simulink model "fourbitserialadder"  (R2023a)
settings: Solver=VariableStepAuto  StartTime=0.0  StopTime=10  RelTol=1e-3
libraries: simulink_extras x12
settings Model: Creator=prath  LastModifiedBy=prath

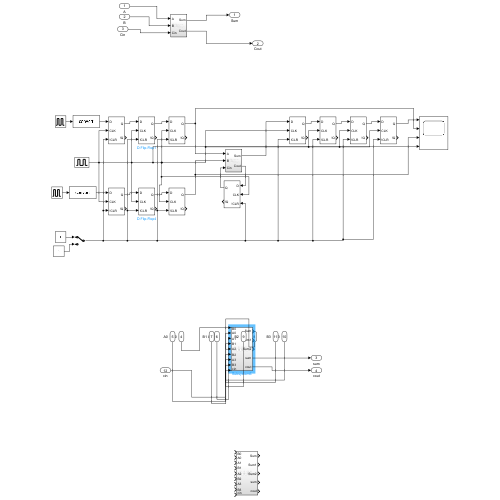
[thumbnail: Simulink's stored preview of the top-level diagram]
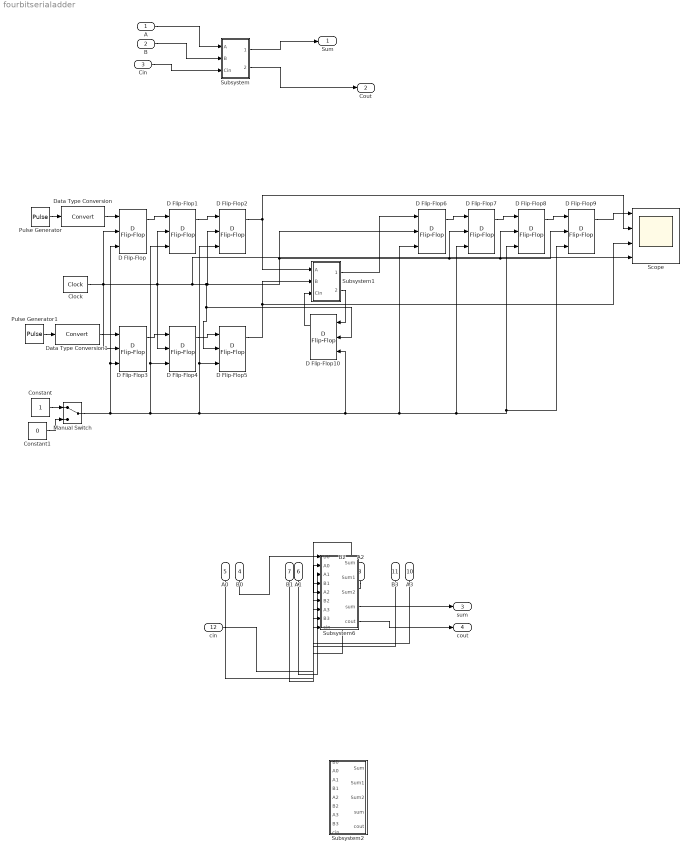
== system fourbitserialadder ==
  A : Inport
  B : Inport  Port=2
  Cin : Inport  Port=3
  B0 : Inport  Port=4
  A0 : Inport  Port=5
  A1 : Inport  Port=6
  B1 : Inport  Port=7
  A2 : Inport  Port=8
  B2 : Inport  Port=9
  A3 : Inport  Port=10
  B3 : Inport  Port=11
  cin : Inport  Port=12
  Clock : simulink_extras/Flip Flops/Clock  period=0.5
  Constant : Constant
  Constant1 : Constant  Value=0
  D Flip-Flop{,1..10} (11 alike) : simulink_extras/Flip Flops/D Flip-Flop
  Data Type Conversion : DataTypeConversion  SaturateOnIntegerOverflow=off  RndMeth=Floor
  Data Type Conversion1 : DataTypeConversion  SaturateOnIntegerOverflow=off  RndMeth=Floor
  Manual Switch : ManualSwitch
  Pulse Generator : DiscretePulseGenerator  PulseType=Time based  PulseWidth=50
  Pulse Generator1 : DiscretePulseGenerator  PulseType=Time based  Period=1  PulseWidth=50
  Scope : Scope  NumInputPorts=4
  Subsystem : Subsystem
  Subsystem1 : Subsystem
  Subsystem2 : Subsystem
  Subsystem6 : Subsystem
  Sum : Outport
  Cout : Outport  Port=2
  sum : Outport  Port=3
  cout : Outport  Port=4
  wires:
  A/1 -> Subsystem/1(A)
  B/1 -> Subsystem/2(B)
  Cin/1 -> Subsystem/3(Cin)
  Subsystem/1(Sum) -> Sum/1
  Subsystem/2(Cout) -> Cout/1
  D Flip-Flop/1 -> D Flip-Flop1/1
  D Flip-Flop1/1 -> D Flip-Flop2/1
  D Flip-Flop3/1 -> D Flip-Flop4/1
  D Flip-Flop4/1 -> D Flip-Flop5/1
  Subsystem1/2(Cout) -> D Flip-Flop10/1
  D Flip-Flop10/1 -> Subsystem1/3(Cin)
  Subsystem1/1(Sum) -> D Flip-Flop6/1
  D Flip-Flop6/1 -> D Flip-Flop7/1
  D Flip-Flop7/1 -> D Flip-Flop8/1
  D Flip-Flop8/1 -> D Flip-Flop9/1
  Clock/1 -> D Flip-Flop3/2, D Flip-Flop4/2, Scope/4, D Flip-Flop9/2, D Flip-Flop8/2, D Flip-Flop7/2, D Flip-Flop6/2, D Flip-Flop2/2, D Flip-Flop10/2, D Flip-Flop5/2, D Flip-Flop1/2, D Flip-Flop/2
  Pulse Generator/1 -> Data Type Conversion/1
  Data Type Conversion/1 -> D Flip-Flop/1
  Pulse Generator1/1 -> Data Type Conversion1/1
  Data Type Conversion1/1 -> D Flip-Flop3/1
  Constant/1 -> Manual Switch/1
  Constant1/1 -> Manual Switch/2
  Manual Switch/1 -> D Flip-Flop3/3, D Flip-Flop/3, D Flip-Flop4/3, D Flip-Flop1/3, D Flip-Flop10/3, D Flip-Flop9/3, D Flip-Flop8/3, D Flip-Flop7/3, D Flip-Flop6/3, D Flip-Flop5/3, D Flip-Flop2/3
  D Flip-Flop2/1 -> Subsystem1/1(A), Scope/2
  D Flip-Flop5/1 -> Scope/3, Subsystem1/2(B)
  D Flip-Flop9/1 -> Scope/1
  B0/1 -> Subsystem6/1(B0)
  A0/1 -> Subsystem6/2(A0)
  A1/1 -> Subsystem6/3(A1)
  B1/1 -> Subsystem6/4(B1)
  A2/1 -> Subsystem6/5(A2)
  B2/1 -> Subsystem6/6(B2)
  A3/1 -> Subsystem6/7(A3)
  B3/1 -> Subsystem6/8(B3)
  cin/1 -> Subsystem6/9(cin)
  Subsystem6/4(sum) -> sum/1
  Subsystem6/5(cout) -> cout/1

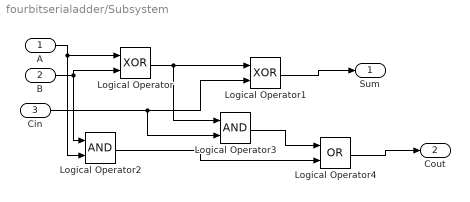
== system fourbitserialadder/Subsystem ==
  A : Inport
  B : Inport  Port=2
  Cin : Inport  Port=3
  Logical Operator : Logic  Operator=XOR  AllPortsSameDT=off  OutDataTypeStr=boolean
  Logical Operator1 : Logic  Operator=XOR  AllPortsSameDT=off  OutDataTypeStr=boolean
  Logical Operator2 : Logic  AllPortsSameDT=off  OutDataTypeStr=boolean
  Logical Operator3 : Logic  AllPortsSameDT=off  OutDataTypeStr=boolean
  Logical Operator4 : Logic  Operator=OR  AllPortsSameDT=off  OutDataTypeStr=boolean
  Sum : Outport
  Cout : Outport  Port=2
  wires:
  B/1 -> Logical Operator/2, Logical Operator2/1
  Cin/1 -> Logical Operator3/2, Logical Operator1/2
  Logical Operator3/1 -> Logical Operator4/1
  Logical Operator2/1 -> Logical Operator4/2
  A/1 -> Logical Operator/1, Logical Operator2/2
  Logical Operator/1 -> Logical Operator3/1, Logical Operator1/1
  Logical Operator1/1 -> Sum/1
  Logical Operator4/1 -> Cout/1

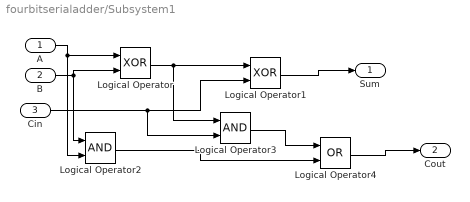
== system fourbitserialadder/Subsystem1 ==
  A : Inport
  B : Inport  Port=2
  Cin : Inport  Port=3
  Logical Operator : Logic  Operator=XOR  AllPortsSameDT=off  OutDataTypeStr=boolean
  Logical Operator1 : Logic  Operator=XOR  AllPortsSameDT=off  OutDataTypeStr=boolean
  Logical Operator2 : Logic  AllPortsSameDT=off  OutDataTypeStr=boolean
  Logical Operator3 : Logic  AllPortsSameDT=off  OutDataTypeStr=boolean
  Logical Operator4 : Logic  Operator=OR  AllPortsSameDT=off  OutDataTypeStr=boolean
  Sum : Outport
  Cout : Outport  Port=2
  wires:
  B/1 -> Logical Operator/2, Logical Operator2/1
  Cin/1 -> Logical Operator3/2, Logical Operator1/2
  Logical Operator3/1 -> Logical Operator4/1
  Logical Operator2/1 -> Logical Operator4/2
  A/1 -> Logical Operator/1, Logical Operator2/2
  Logical Operator/1 -> Logical Operator3/1, Logical Operator1/1
  Logical Operator1/1 -> Sum/1
  Logical Operator4/1 -> Cout/1

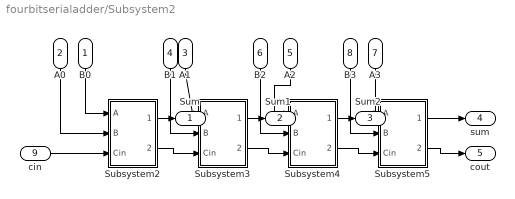
== system fourbitserialadder/Subsystem2 ==
  B0 : Inport
  A0 : Inport  Port=2
  A1 : Inport  Port=3
  B1 : Inport  Port=4
  A2 : Inport  Port=5
  B2 : Inport  Port=6
  A3 : Inport  Port=7
  B3 : Inport  Port=8
  cin : Inport  Port=9
  Subsystem2 : Subsystem
  Subsystem3 : Subsystem
  Subsystem4 : Subsystem
  Subsystem5 : Subsystem
  Sum : Outport
  Sum1 : Outport  Port=2
  Sum2 : Outport  Port=3
  sum : Outport  Port=4
  cout : Outport  Port=5
  wires:
  B0/1 -> Subsystem2/1(A)
  A2/1 -> Subsystem4/1(A)
  Subsystem2/1(Sum) -> Sum/1
  A3/1 -> Subsystem5/1(A)
  Subsystem4/1(Sum) -> Sum2/1
  cin/1 -> Subsystem2/3(Cin)
  B1/1 -> Subsystem3/2(B)
  Subsystem5/1(Sum) -> sum/1
  B2/1 -> Subsystem4/2(B)
  Subsystem5/2(Cout) -> cout/1
  B3/1 -> Subsystem5/2(B)
  Subsystem2/2(Cout) -> Subsystem3/3(Cin)
  Subsystem3/2(Cout) -> Subsystem4/3(Cin)
  Subsystem4/2(Cout) -> Subsystem5/3(Cin)
  A1/1 -> Subsystem3/1(A)
  A0/1 -> Subsystem2/2(B)
  Subsystem3/1(Sum) -> Sum1/1

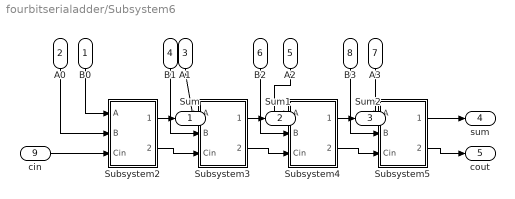
== system fourbitserialadder/Subsystem6 ==
  B0 : Inport
  A0 : Inport  Port=2
  A1 : Inport  Port=3
  B1 : Inport  Port=4
  A2 : Inport  Port=5
  B2 : Inport  Port=6
  A3 : Inport  Port=7
  B3 : Inport  Port=8
  cin : Inport  Port=9
  Subsystem2 : Subsystem
  Subsystem3 : Subsystem
  Subsystem4 : Subsystem
  Subsystem5 : Subsystem
  Sum : Outport
  Sum1 : Outport  Port=2
  Sum2 : Outport  Port=3
  sum : Outport  Port=4
  cout : Outport  Port=5
  wires:
  B0/1 -> Subsystem2/1(A)
  A2/1 -> Subsystem4/1(A)
  Subsystem2/1(Sum) -> Sum/1
  A3/1 -> Subsystem5/1(A)
  Subsystem4/1(Sum) -> Sum2/1
  cin/1 -> Subsystem2/3(Cin)
  B1/1 -> Subsystem3/2(B)
  Subsystem5/1(Sum) -> sum/1
  B2/1 -> Subsystem4/2(B)
  Subsystem5/2(Cout) -> cout/1
  B3/1 -> Subsystem5/2(B)
  Subsystem2/2(Cout) -> Subsystem3/3(Cin)
  Subsystem3/2(Cout) -> Subsystem4/3(Cin)
  Subsystem4/2(Cout) -> Subsystem5/3(Cin)
  A1/1 -> Subsystem3/1(A)
  A0/1 -> Subsystem2/2(B)
  Subsystem3/1(Sum) -> Sum1/1

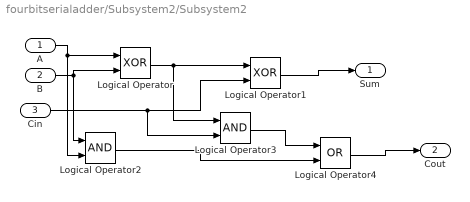
== system fourbitserialadder/Subsystem2/Subsystem2 ==
  A : Inport
  B : Inport  Port=2
  Cin : Inport  Port=3
  Logical Operator : Logic  Operator=XOR  AllPortsSameDT=off  OutDataTypeStr=boolean
  Logical Operator1 : Logic  Operator=XOR  AllPortsSameDT=off  OutDataTypeStr=boolean
  Logical Operator2 : Logic  AllPortsSameDT=off  OutDataTypeStr=boolean
  Logical Operator3 : Logic  AllPortsSameDT=off  OutDataTypeStr=boolean
  Logical Operator4 : Logic  Operator=OR  AllPortsSameDT=off  OutDataTypeStr=boolean
  Sum : Outport
  Cout : Outport  Port=2
  wires:
  B/1 -> Logical Operator/2, Logical Operator2/1
  Cin/1 -> Logical Operator3/2, Logical Operator1/2
  Logical Operator3/1 -> Logical Operator4/1
  Logical Operator2/1 -> Logical Operator4/2
  A/1 -> Logical Operator/1, Logical Operator2/2
  Logical Operator/1 -> Logical Operator3/1, Logical Operator1/1
  Logical Operator1/1 -> Sum/1
  Logical Operator4/1 -> Cout/1

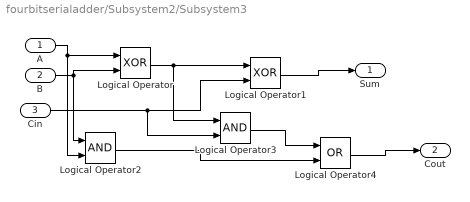
== system fourbitserialadder/Subsystem2/Subsystem3 ==
  A : Inport
  B : Inport  Port=2
  Cin : Inport  Port=3
  Logical Operator : Logic  Operator=XOR  AllPortsSameDT=off  OutDataTypeStr=boolean
  Logical Operator1 : Logic  Operator=XOR  AllPortsSameDT=off  OutDataTypeStr=boolean
  Logical Operator2 : Logic  AllPortsSameDT=off  OutDataTypeStr=boolean
  Logical Operator3 : Logic  AllPortsSameDT=off  OutDataTypeStr=boolean
  Logical Operator4 : Logic  Operator=OR  AllPortsSameDT=off  OutDataTypeStr=boolean
  Sum : Outport
  Cout : Outport  Port=2
  wires:
  B/1 -> Logical Operator/2, Logical Operator2/1
  Cin/1 -> Logical Operator3/2, Logical Operator1/2
  Logical Operator3/1 -> Logical Operator4/1
  Logical Operator2/1 -> Logical Operator4/2
  A/1 -> Logical Operator/1, Logical Operator2/2
  Logical Operator/1 -> Logical Operator3/1, Logical Operator1/1
  Logical Operator1/1 -> Sum/1
  Logical Operator4/1 -> Cout/1

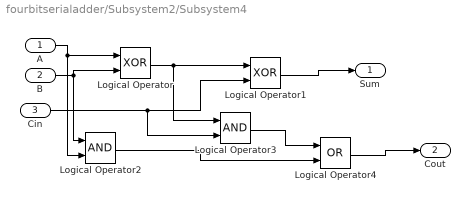
== system fourbitserialadder/Subsystem2/Subsystem4 ==
  A : Inport
  B : Inport  Port=2
  Cin : Inport  Port=3
  Logical Operator : Logic  Operator=XOR  AllPortsSameDT=off  OutDataTypeStr=boolean
  Logical Operator1 : Logic  Operator=XOR  AllPortsSameDT=off  OutDataTypeStr=boolean
  Logical Operator2 : Logic  AllPortsSameDT=off  OutDataTypeStr=boolean
  Logical Operator3 : Logic  AllPortsSameDT=off  OutDataTypeStr=boolean
  Logical Operator4 : Logic  Operator=OR  AllPortsSameDT=off  OutDataTypeStr=boolean
  Sum : Outport
  Cout : Outport  Port=2
  wires:
  B/1 -> Logical Operator/2, Logical Operator2/1
  Cin/1 -> Logical Operator3/2, Logical Operator1/2
  Logical Operator3/1 -> Logical Operator4/1
  Logical Operator2/1 -> Logical Operator4/2
  A/1 -> Logical Operator/1, Logical Operator2/2
  Logical Operator/1 -> Logical Operator3/1, Logical Operator1/1
  Logical Operator1/1 -> Sum/1
  Logical Operator4/1 -> Cout/1

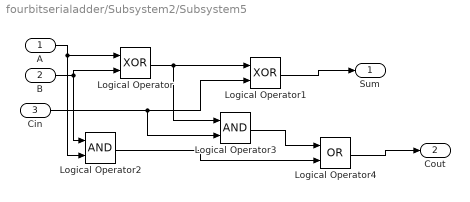
== system fourbitserialadder/Subsystem2/Subsystem5 ==
  A : Inport
  B : Inport  Port=2
  Cin : Inport  Port=3
  Logical Operator : Logic  Operator=XOR  AllPortsSameDT=off  OutDataTypeStr=boolean
  Logical Operator1 : Logic  Operator=XOR  AllPortsSameDT=off  OutDataTypeStr=boolean
  Logical Operator2 : Logic  AllPortsSameDT=off  OutDataTypeStr=boolean
  Logical Operator3 : Logic  AllPortsSameDT=off  OutDataTypeStr=boolean
  Logical Operator4 : Logic  Operator=OR  AllPortsSameDT=off  OutDataTypeStr=boolean
  Sum : Outport
  Cout : Outport  Port=2
  wires:
  B/1 -> Logical Operator/2, Logical Operator2/1
  Cin/1 -> Logical Operator3/2, Logical Operator1/2
  Logical Operator3/1 -> Logical Operator4/1
  Logical Operator2/1 -> Logical Operator4/2
  A/1 -> Logical Operator/1, Logical Operator2/2
  Logical Operator/1 -> Logical Operator3/1, Logical Operator1/1
  Logical Operator1/1 -> Sum/1
  Logical Operator4/1 -> Cout/1

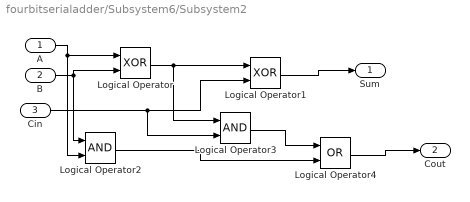
== system fourbitserialadder/Subsystem6/Subsystem2 ==
  A : Inport
  B : Inport  Port=2
  Cin : Inport  Port=3
  Logical Operator : Logic  Operator=XOR  AllPortsSameDT=off  OutDataTypeStr=boolean
  Logical Operator1 : Logic  Operator=XOR  AllPortsSameDT=off  OutDataTypeStr=boolean
  Logical Operator2 : Logic  AllPortsSameDT=off  OutDataTypeStr=boolean
  Logical Operator3 : Logic  AllPortsSameDT=off  OutDataTypeStr=boolean
  Logical Operator4 : Logic  Operator=OR  AllPortsSameDT=off  OutDataTypeStr=boolean
  Sum : Outport
  Cout : Outport  Port=2
  wires:
  B/1 -> Logical Operator/2, Logical Operator2/1
  Cin/1 -> Logical Operator3/2, Logical Operator1/2
  Logical Operator3/1 -> Logical Operator4/1
  Logical Operator2/1 -> Logical Operator4/2
  A/1 -> Logical Operator/1, Logical Operator2/2
  Logical Operator/1 -> Logical Operator3/1, Logical Operator1/1
  Logical Operator1/1 -> Sum/1
  Logical Operator4/1 -> Cout/1

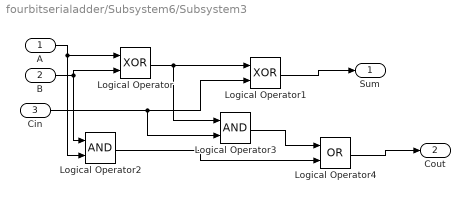
== system fourbitserialadder/Subsystem6/Subsystem3 ==
  A : Inport
  B : Inport  Port=2
  Cin : Inport  Port=3
  Logical Operator : Logic  Operator=XOR  AllPortsSameDT=off  OutDataTypeStr=boolean
  Logical Operator1 : Logic  Operator=XOR  AllPortsSameDT=off  OutDataTypeStr=boolean
  Logical Operator2 : Logic  AllPortsSameDT=off  OutDataTypeStr=boolean
  Logical Operator3 : Logic  AllPortsSameDT=off  OutDataTypeStr=boolean
  Logical Operator4 : Logic  Operator=OR  AllPortsSameDT=off  OutDataTypeStr=boolean
  Sum : Outport
  Cout : Outport  Port=2
  wires:
  B/1 -> Logical Operator/2, Logical Operator2/1
  Cin/1 -> Logical Operator3/2, Logical Operator1/2
  Logical Operator3/1 -> Logical Operator4/1
  Logical Operator2/1 -> Logical Operator4/2
  A/1 -> Logical Operator/1, Logical Operator2/2
  Logical Operator/1 -> Logical Operator3/1, Logical Operator1/1
  Logical Operator1/1 -> Sum/1
  Logical Operator4/1 -> Cout/1

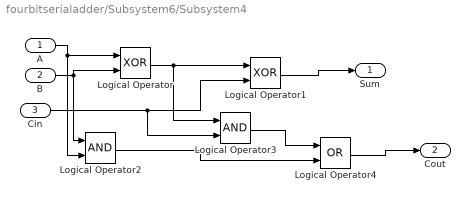
== system fourbitserialadder/Subsystem6/Subsystem4 ==
  A : Inport
  B : Inport  Port=2
  Cin : Inport  Port=3
  Logical Operator : Logic  Operator=XOR  AllPortsSameDT=off  OutDataTypeStr=boolean
  Logical Operator1 : Logic  Operator=XOR  AllPortsSameDT=off  OutDataTypeStr=boolean
  Logical Operator2 : Logic  AllPortsSameDT=off  OutDataTypeStr=boolean
  Logical Operator3 : Logic  AllPortsSameDT=off  OutDataTypeStr=boolean
  Logical Operator4 : Logic  Operator=OR  AllPortsSameDT=off  OutDataTypeStr=boolean
  Sum : Outport
  Cout : Outport  Port=2
  wires:
  B/1 -> Logical Operator/2, Logical Operator2/1
  Cin/1 -> Logical Operator3/2, Logical Operator1/2
  Logical Operator3/1 -> Logical Operator4/1
  Logical Operator2/1 -> Logical Operator4/2
  A/1 -> Logical Operator/1, Logical Operator2/2
  Logical Operator/1 -> Logical Operator3/1, Logical Operator1/1
  Logical Operator1/1 -> Sum/1
  Logical Operator4/1 -> Cout/1

== system fourbitserialadder/Subsystem6/Subsystem5 ==
  A : Inport
  B : Inport  Port=2
  Cin : Inport  Port=3
  Logical Operator : Logic  Operator=XOR  AllPortsSameDT=off  OutDataTypeStr=boolean
  Logical Operator1 : Logic  Operator=XOR  AllPortsSameDT=off  OutDataTypeStr=boolean
  Logical Operator2 : Logic  AllPortsSameDT=off  OutDataTypeStr=boolean
  Logical Operator3 : Logic  AllPortsSameDT=off  OutDataTypeStr=boolean
  Logical Operator4 : Logic  Operator=OR  AllPortsSameDT=off  OutDataTypeStr=boolean
  Sum : Outport
  Cout : Outport  Port=2
  wires:
  B/1 -> Logical Operator/2, Logical Operator2/1
  Cin/1 -> Logical Operator3/2, Logical Operator1/2
  Logical Operator3/1 -> Logical Operator4/1
  Logical Operator2/1 -> Logical Operator4/2
  A/1 -> Logical Operator/1, Logical Operator2/2
  Logical Operator/1 -> Logical Operator3/1, Logical Operator1/1
  Logical Operator1/1 -> Sum/1
  Logical Operator4/1 -> Cout/1
